simulink library "lib_rfsignalgenerator"  (R2022a)
settings: Solver=VariableStepAuto  StartTime=0.0  StopTime=10.0  RelTol=1e-3
undefined symbols (not defined in the file or in its folder): fs, QAM1024_Sym, QAM512_Sym
libraries: hdlsllib x41, simulink x15, commseqgen3 x10
(part 2 of 2)

== system lib_rfsignalgenerator/RF Signal Generator/Variable Modulator/QAM32 Generator/complement_im ==
  d_in : Inport
  Add : Sum  OutDataTypeStr=uint16
  Bitwise NOT : simulink/Logic and Bit Operations/Bitwise Operator  logicop=NOT  UseBitMask=off  BitMask=bin2dec('11011001')  BitMaskRealWorld=Stored Integer
  Constant1 : Constant  OutDataTypeStr=uint16  SampleTime=1/fs
  Data Type Conversion : DataTypeConversion  OutDataTypeStr=uint16  ConvertRealWorld=Stored Integer (SI)  SaturateOnIntegerOverflow=off  RndMeth=Floor
  Data Type Conversion1 : DataTypeConversion  OutDataTypeStr=fixdt(1,16,14)  ConvertRealWorld=Stored Integer (SI)  SaturateOnIntegerOverflow=off  RndMeth=Floor
  d_out : Outport
  wires:
  Data Type Conversion1/1 -> d_out/1
  Data Type Conversion/1 -> Bitwise NOT/1
  Constant1/1 -> Add/2
  Bitwise NOT/1 -> Add/1
  d_in/1 -> Data Type Conversion/1
  Add/1 -> Data Type Conversion1/1

== system lib_rfsignalgenerator/RF Signal Generator/Variable Modulator/QAM32 Generator/complement_re ==
  d_in : Inport
  Add : Sum  OutDataTypeStr=uint16
  Bitwise NOT : simulink/Logic and Bit Operations/Bitwise Operator  logicop=NOT  UseBitMask=off  BitMask=bin2dec('11011001')  BitMaskRealWorld=Stored Integer
  Constant1 : Constant  OutDataTypeStr=uint16  SampleTime=1/fs
  Data Type Conversion : DataTypeConversion  OutDataTypeStr=uint16  ConvertRealWorld=Stored Integer (SI)  SaturateOnIntegerOverflow=off  RndMeth=Floor
  Data Type Conversion1 : DataTypeConversion  OutDataTypeStr=fixdt(1,16,14)  ConvertRealWorld=Stored Integer (SI)  SaturateOnIntegerOverflow=off  RndMeth=Floor
  d_out : Outport
  wires:
  Add/1 -> Data Type Conversion1/1
  d_in/1 -> Data Type Conversion/1
  Bitwise NOT/1 -> Add/1
  Constant1/1 -> Add/2
  Data Type Conversion/1 -> Bitwise NOT/1
  Data Type Conversion1/1 -> d_out/1

== system lib_rfsignalgenerator/RF Signal Generator/Variable Modulator/QAM512 Generator/complement2 ==
  d_in : Inport
  Add : Sum  OutDataTypeStr=uint16
  Bitwise NOT : simulink/Logic and Bit Operations/Bitwise Operator  logicop=NOT  UseBitMask=off  BitMask=bin2dec('11011001')  BitMaskRealWorld=Stored Integer
  Constant1 : Constant  OutDataTypeStr=uint16  SampleTime=1/fs
  Data Type Conversion : DataTypeConversion  OutDataTypeStr=uint16  ConvertRealWorld=Stored Integer (SI)  SaturateOnIntegerOverflow=off  RndMeth=Floor
  Data Type Conversion1 : DataTypeConversion  OutDataTypeStr=fixdt(1,16,14)  ConvertRealWorld=Stored Integer (SI)  SaturateOnIntegerOverflow=off  RndMeth=Floor
  d_out : Outport
  wires:
  Add/1 -> Data Type Conversion1/1
  d_in/1 -> Data Type Conversion/1
  Bitwise NOT/1 -> Add/1
  Constant1/1 -> Add/2
  Data Type Conversion/1 -> Bitwise NOT/1
  Data Type Conversion1/1 -> d_out/1

== system lib_rfsignalgenerator/RF Signal Generator/Variable Modulator/QAM512 Generator/complement_im2 ==
  d_in : Inport
  Add : Sum  OutDataTypeStr=uint16
  Bitwise NOT : simulink/Logic and Bit Operations/Bitwise Operator  logicop=NOT  UseBitMask=off  BitMask=bin2dec('11011001')  BitMaskRealWorld=Stored Integer
  Constant1 : Constant  OutDataTypeStr=uint16  SampleTime=1/fs
  Data Type Conversion : DataTypeConversion  OutDataTypeStr=uint16  ConvertRealWorld=Stored Integer (SI)  SaturateOnIntegerOverflow=off  RndMeth=Floor
  Data Type Conversion1 : DataTypeConversion  OutDataTypeStr=fixdt(1,16,14)  ConvertRealWorld=Stored Integer (SI)  SaturateOnIntegerOverflow=off  RndMeth=Floor
  d_out : Outport
  wires:
  Add/1 -> Data Type Conversion1/1
  d_in/1 -> Data Type Conversion/1
  Bitwise NOT/1 -> Add/1
  Constant1/1 -> Add/2
  Data Type Conversion/1 -> Bitwise NOT/1
  Data Type Conversion1/1 -> d_out/1

== system lib_rfsignalgenerator/RF Signal Generator/Variable Modulator/QAM512 Generator/complement_re ==
  d_in : Inport
  Add : Sum  OutDataTypeStr=uint16
  Bitwise NOT : simulink/Logic and Bit Operations/Bitwise Operator  logicop=NOT  UseBitMask=off  BitMask=bin2dec('11011001')  BitMaskRealWorld=Stored Integer
  Constant1 : Constant  OutDataTypeStr=uint16  SampleTime=1/fs
  Data Type Conversion : DataTypeConversion  OutDataTypeStr=uint16  ConvertRealWorld=Stored Integer (SI)  SaturateOnIntegerOverflow=off  RndMeth=Floor
  Data Type Conversion1 : DataTypeConversion  OutDataTypeStr=fixdt(1,16,14)  ConvertRealWorld=Stored Integer (SI)  SaturateOnIntegerOverflow=off  RndMeth=Floor
  d_out : Outport
  wires:
  Data Type Conversion1/1 -> d_out/1
  Data Type Conversion/1 -> Bitwise NOT/1
  Constant1/1 -> Add/2
  Bitwise NOT/1 -> Add/1
  d_in/1 -> Data Type Conversion/1
  Add/1 -> Data Type Conversion1/1

== system lib_rfsignalgenerator/RF Signal Generator/Variable Modulator/QAM64 Generator/complement_im ==
  d_in : Inport
  Add : Sum  OutDataTypeStr=uint16
  Bitwise NOT : simulink/Logic and Bit Operations/Bitwise Operator  logicop=NOT  UseBitMask=off  BitMask=bin2dec('11011001')  BitMaskRealWorld=Stored Integer
  Constant1 : Constant  OutDataTypeStr=uint16  SampleTime=1/fs
  Data Type Conversion : DataTypeConversion  OutDataTypeStr=uint16  ConvertRealWorld=Stored Integer (SI)  SaturateOnIntegerOverflow=off  RndMeth=Floor
  Data Type Conversion1 : DataTypeConversion  OutDataTypeStr=fixdt(1,16,14)  ConvertRealWorld=Stored Integer (SI)  SaturateOnIntegerOverflow=off  RndMeth=Floor
  d_out : Outport
  wires:
  Add/1 -> Data Type Conversion1/1
  d_in/1 -> Data Type Conversion/1
  Bitwise NOT/1 -> Add/1
  Constant1/1 -> Add/2
  Data Type Conversion/1 -> Bitwise NOT/1
  Data Type Conversion1/1 -> d_out/1

== system lib_rfsignalgenerator/RF Signal Generator/Variable Modulator/QAM64 Generator/complement_re ==
  d_in : Inport
  Add : Sum  OutDataTypeStr=uint16
  Bitwise NOT : simulink/Logic and Bit Operations/Bitwise Operator  logicop=NOT  UseBitMask=off  BitMask=bin2dec('11011001')  BitMaskRealWorld=Stored Integer
  Constant1 : Constant  OutDataTypeStr=uint16  SampleTime=1/fs
  Data Type Conversion : DataTypeConversion  OutDataTypeStr=uint16  ConvertRealWorld=Stored Integer (SI)  SaturateOnIntegerOverflow=off  RndMeth=Floor
  Data Type Conversion1 : DataTypeConversion  OutDataTypeStr=fixdt(1,16,14)  ConvertRealWorld=Stored Integer (SI)  SaturateOnIntegerOverflow=off  RndMeth=Floor
  d_out : Outport
  wires:
  Data Type Conversion1/1 -> d_out/1
  Data Type Conversion/1 -> Bitwise NOT/1
  Constant1/1 -> Add/2
  Bitwise NOT/1 -> Add/1
  d_in/1 -> Data Type Conversion/1
  Add/1 -> Data Type Conversion1/1
